simulink model "sim_new_traj_only_att_ctrl"  (R2020a)
settings: Solver=ode4  StartTime=0.0  StopTime=30.0  FixedStep=0.01  RelTol=1e-3
values from neighbouring files (symbols this model uses):
  beta_Phi_1 = pp0 * cal_frac_squ( 3, p_p0_plus_1, q_p0_plus_1 )                          * cal_frac_squ( eps_s_bar / pi, p_p0_min_2, q_p0_min_2 )                          / ( 2 * ( 2 * pp0 - 1 ) * tanh( gamma0 * ( eps_s_bar / pi ) / 2 ) )                          - ( cal_frac_squ( 3, p_p0_plus_1, q_p0_plus_1 ) * gamma0 / ( 4 * ( 2 * pp0 -1 ) ) )                          * cal_frac_squ( eps_s_bar / pi, p_p0_min_ ...(+136 chars)    [init_new_traj_only_att_ctrl.m]
  beta_Phi_2 = ( 1 - pp0 ) * cal_frac_squ( 3, p_p0_plus_1, q_p0_plus_1 )                          / ( 2 * ( 1 - 2 * pp0 ) * cal_frac_squ( eps_s_bar / pi, p_p0_0, q_p0_0 ) * tanh( gamma0 * ( eps_s_bar / pi ) / 2 ) )                          - ( cal_frac_squ( 3, p_p0_plus_1, q_p0_plus_1 ) * gamma0 / ( 4 * ( 1 - 2 * pp0 ) ) )                          * cal_frac_squ( eps_s_bar / pi, p_1_min_p0, q_1_min_p0 )          ...(+112 chars)    [init_new_traj_only_att_ctrl.m]
  c1_diff_sigma_bar_w = diag([12; 12; 12])    [init_new_traj_only_att_ctrl.m]
  c1_diff_ui = diag([25; 30; 20])    [init_new_traj_only_att_ctrl.m]
  c2_diff_sigma_bar_w = diag([12; 12; 12])    [init_new_traj_only_att_ctrl.m]
  c2_diff_ui = diag([50; 50; 10])    [init_new_traj_only_att_ctrl.m]
  c3_diff_sigma_bar_w = diag([15; 15; 15])    [init_new_traj_only_att_ctrl.m]
  c3_diff_ui = diag([15; 15; 10])    [init_new_traj_only_att_ctrl.m]
  c_w_1 = diag( [20; 15; 15] )    [init_new_traj_only_att_ctrl.m]
  c_w_2 = diag( [20; 15; 15] )    [init_new_traj_only_att_ctrl.m]
  c_w_3 = diag( [2; 2; 2] )    [init_new_traj_only_att_ctrl.m]
  cS0 = diag( [4.5; 4.5; 4.5] )    [init_new_traj_only_att_ctrl.m]
  dw_aa_t = 0.2 * ones(3, 5) + ( 1.0 - 0.2 ) * rand(3, 5)    [init_new_traj_only_att_ctrl.m]
  dw_ff_t = [ 0.4 * ones(1, 5) + ( 1.0 - 0.4 ) * rand(1, 5);                      0.4 * ones(1, 5) + ( 1.0 - 0.4 ) * rand(1, 5);                      0.2 * ones(1, 5) + ( 0.6 - 0.2 ) * rand(1, 5) ]    [init_new_traj_only_att_ctrl.m]
  dw_phi_t = ( - pi / 2 ) * ones(3, 5) + ( pi / 2 - ( - pi / 2 ) ) * rand(3, 5)    [init_new_traj_only_att_ctrl.m]
  dwci_init = zeros(3,5)    [init_new_traj_only_att_ctrl.m]
  eps_s_bar_div_pi = eps_s_bar / pi    (= 0.03)    [init_new_traj_only_att_ctrl.m]
  gamma0 = 20    [init_new_traj_only_att_ctrl.m]
  h1w = diag([20.0; 20.0; 20.0])    [init_new_traj_only_att_ctrl.m]
  h2w = diag([30.0; 35.0; 35.0])    [init_new_traj_only_att_ctrl.m]
  h3w = diag([30.0; 25.0; 30.0])    [init_new_traj_only_att_ctrl.m]
  Ji = zeros(3,3,NF)    [init_new_traj_only_att_ctrl.m]
  k_J_0 = diag( [1; 1; 1] )    [init_new_traj_only_att_ctrl.m]
  Lamd_diff_sigma_bar_w = 0.8    [init_new_traj_only_att_ctrl.m]
  Lamd_diff_ui = 0.8    [init_new_traj_only_att_ctrl.m]
  mu_c_theta = 100    [init_new_traj_only_att_ctrl.m]
  mu_d_w = 100    [init_new_traj_only_att_ctrl.m]
  pos0 = zeros(3, 1)    [init_new_traj_only_att_ctrl.m]
  pp0 = 8 / 11    (= 0.727272727273)    [init_new_traj_only_att_ctrl.m]
  PZ0 = P0(3)    [init_new_traj_only_att_ctrl.m]
  PZ1 = 10    [init_new_traj_only_att_ctrl.m]
  Qci_init = repmat([1;0;0;0],1,NF)    [init_new_traj_only_att_ctrl.m]
  R0 = 4    [init_new_traj_only_att_ctrl.m]
  R1 = 8    [init_new_traj_only_att_ctrl.m]
  Rci_init = zeros(3,3,NF)    [init_new_traj_only_att_ctrl.m]
  Ri_init = zeros(3,3,NF)    [init_new_traj_only_att_ctrl.m]
  Rx2 = 10    [init_new_traj_only_att_ctrl.m]
  Ry2 = 6    [init_new_traj_only_att_ctrl.m]
  Rz2 = 4    [init_new_traj_only_att_ctrl.m]
  T0 = 0    [init_new_traj_only_att_ctrl.m]
  T1 = tseq1    (= 10)    [init_new_traj_only_att_ctrl.m]
  T2 = tseq1 + tseq12 + tseq2    (= 30)    [init_new_traj_only_att_ctrl.m]
  thr_p_plus_1 = cal_frac_squ( 3, p_p0_plus_1, q_p0_plus_1 )    [init_new_traj_only_att_ctrl.m]
  ui_init = zeros(3,NF)    [init_new_traj_only_att_ctrl.m]
  vel0 = zeros(3, 1)    [init_new_traj_only_att_ctrl.m]
  wci_init = zeros(3,5)    [init_new_traj_only_att_ctrl.m]
  zeta_diff_sigma_bar_w = 0.3    [init_new_traj_only_att_ctrl.m]
  zeta_diff_ui = 0.05    [init_new_traj_only_att_ctrl.m]
undefined symbols (not defined in the file or in its folder): cal_frac_squ, p_2_p0, p_alfaw1, p_alfaw2, p_beta_w_1, p_beta_w_2, p_p0_min_1, p_p0_plus_1, q_2_p0, q_alfaw1, q_alfaw2, q_beta_w_1, q_beta_w_2, q_p0_min_1, q_p0_plus_1, Qei_init, Qi_init, Rei_init, V_Phi_Rei_init, wei_init, wi_init
(part 2 of 5)

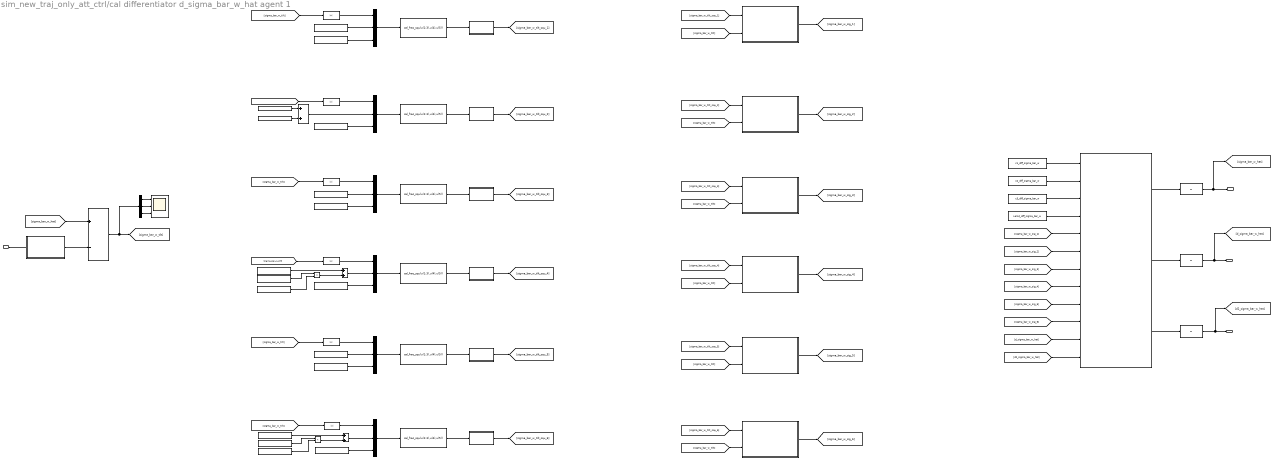
== system sim_new_traj_only_att_ctrl/cal differentiator d_sigma_bar_w_hat agent 1 ==
  x : Inport
  Abs{,1..5} (6 alike) : Abs
  Add : Sum
  Add1 : Sum
  Add2 : Sum
  Add3 : Sum  Inputs=+-
  Constant : Constant  Value=0
  Constant{97,100,105,107,109} (5 alike) : Constant
  Constant{98..99,101,108,110..111} (6 alike) : Constant  Value=3
  Constant102 : Constant  Value=2
  Constant103 : Constant  Value=c1_diff_sigma_bar_w
  Constant104 : Constant  Value=c2_diff_sigma_bar_w
  Constant106 : Constant  Value=c3_diff_sigma_bar_w
  Constant112 : Constant  Value=2
  Constant113 : Constant  Value=Lamd_diff_sigma_bar_w
  Constant161 : Constant  Value=zeta_diff_sigma_bar_w
  Constant162 : Constant  Value=zeta_diff_sigma_bar_w
  Constant163 : Constant  Value=zeta_diff_sigma_bar_w
  Demux2 : Demux  Outputs=3
  Integrator2 : Integrator  InitialCondition=zeros(3,1)
  Integrator3 : Integrator  InitialCondition=zeros(3,1)
  Integrator4 : Integrator  InitialCondition=zeros(3,1)
  Interpreted MATLAB Function{,20..24} (6 alike) : MATLABFcn  MATLABFcn=cal_frac_squ(u(1:3),u(4),u(5))
  Mux{19..24} (6 alike) : Mux  Inputs=3
  Product : Product
  Product1 : Product
  cal differentiator : MATLAB Function  TreatAsAtomicUnit=on
  cal sig : MATLAB Function  TreatAsAtomicUnit=on
  cal sig1 : MATLAB Function  TreatAsAtomicUnit=on
  cal sig2 : MATLAB Function  TreatAsAtomicUnit=on
  cal sig3 : MATLAB Function  TreatAsAtomicUnit=on
  cal sig4 : MATLAB Function  TreatAsAtomicUnit=on
  cal sig5 : MATLAB Function  TreatAsAtomicUnit=on
  choose sigma_bar_w : MATLAB Function  TreatAsAtomicUnit=on
  sigma_bar_w_tilt : Scope  NumInputPorts=3
  trans to column20 : MATLAB Function  TreatAsAtomicUnit=on
  trans to column21 : MATLAB Function  TreatAsAtomicUnit=on
  trans to column22 : MATLAB Function  TreatAsAtomicUnit=on
  trans to column23 : MATLAB Function  TreatAsAtomicUnit=on
  trans to column24 : MATLAB Function  TreatAsAtomicUnit=on
  trans to column25 : MATLAB Function  TreatAsAtomicUnit=on
  Out1 : Outport
  Out2 : Outport  Port=2
  Out3 : Outport  Port=3
  wires:
  Abs/1 -> Mux22/1
  [sigma_bar_w_tilt] -> cal sig/2(y)
  cal sig1/1(z) -> [sigma_bar_w_sig_2]
  [d2_sigma_bar_w_hat] -> cal differentiator/12(d2_sigma_bar_v_hat)
  trans to column23/1(y) -> [sigma_bar_w_tilt_squ_3]
  Add/1 -> Mux21/2
  Demux2/1 -> sigma_bar_w_tilt/1
  [sigma_bar_w_tilt] -> cal sig4/2(y)
  Product1/1 -> Add2/2
  Add2/1 -> Mux19/2
  [d_sigma_bar_w_hat] -> cal differentiator/11("d_sigma_bar_v_hat ")
  [sigma_bar_w_sig_3] -> cal differentiator/7(sigma_bar_v_sig_3)
  trans to column24/1(y) -> [sigma_bar_w_tilt_squ_4]
  Constant107/1 -> Mux21/3
  [sigma_bar_w_sig_5] -> cal differentiator/9(sigma_bar_v_sig_5)
  Constant97/1 -> Mux22/3
  cal sig/1(z) -> [sigma_bar_w_sig_1]
  trans to column22/1(y) -> [sigma_bar_w_tilt_squ_1]
  [sigma_bar_w_tilt_squ_3] -> cal sig2/1(x)
  [sigma_bar_w_tilt] -> Abs3/1
  Interpreted MATLAB Function24/1 -> trans to column25/1(x)
  [sigma_bar_w_sig_1] -> cal differentiator/5(sigma_bar_v_sig_1)
  cal differentiator/1(d_sigma_bar_v_hat) -> Integrator2/1
  Constant110/1 -> Mux24/3
  cal sig5/1(z) -> [sigma_bar_w_sig_5]
  [sigma_bar_w_tilt] -> Abs4/1
  Demux2/3 -> sigma_bar_w_tilt/3
  cal sig2/1(z) -> [sigma_bar_w_sig_3]
  Constant112/1 -> Product/1
  Constant/1 -> Mux22/2
  cal differentiator/3(d_d2sigma_bar_v_hat) -> Integrator4/1
  Abs3/1 -> Mux24/1
  trans to column21/1(y) -> [sigma_bar_w_tilt_squ_2]
  Constant99/1 -> Add2/1
  Constant103/1 -> cal differentiator/1(c1)
  Mux19/1 -> Interpreted MATLAB Function24/1
  [sigma_bar_w_tilt_squ_6] -> cal sig3/1(x)
  Constant106/1 -> cal differentiator/3(c3)
  [sigma_bar_w_tilt] -> Abs2/1
  [sigma_bar_w_tilt_squ_2] -> cal sig1/1(x)
  Constant162/1 -> Product/2
  Product/1 -> Add1/2
  [sigma_bar_w_sig_4] -> cal differentiator/8(sigma_bar_v_sig_4)
  [sigma_bar_w_hat] -> Add3/1
  Constant102/1 -> Mux20/2
  Add3/1 -> Demux2/1, [sigma_bar_w_tilt]
  cal differentiator/2(d_dsigma_bar_v_hat) -> Integrator3/1
  [sigma_bar_w_tilt] -> Abs5/1
  [sigma_bar_w_tilt] -> cal sig2/2(y)
  [sigma_bar_w_sig_6] -> cal differentiator/10(sigma_bar_v_sig_6)
  trans to column20/1(y) -> [sigma_bar_w_tilt_squ_5]
  Constant104/1 -> cal differentiator/2(c2)
  Constant101/1 -> Mux20/3
  Mux22/1 -> Interpreted MATLAB Function/1
  Constant163/1 -> Product1/2
  Abs2/1 -> Mux23/1
  Interpreted MATLAB Function21/1 -> trans to column21/1(x)
  Interpreted MATLAB Function23/1 -> trans to column24/1(x)
  Mux23/1 -> Interpreted MATLAB Function22/1
  cal sig3/1(z) -> [sigma_bar_w_sig_6]
  Abs4/1 -> Mux19/1
  trans to column25/1(y) -> [sigma_bar_w_tilt_squ_6]
  Constant113/1 -> cal differentiator/4(chi_t)
  choose sigma_bar_w/1(y) -> Add3/2
  Interpreted MATLAB Function/1 -> trans to column22/1(x)
  Interpreted MATLAB Function20/1 -> trans to column20/1(x)
  Constant108/1 -> Mux23/3
  [sigma_bar_w_sig_2] -> cal differentiator/6(sigma_bar_v_sig_2)
  [sigma_bar_w_tilt] -> cal sig1/2(y)
  [sigma_bar_w_tilt_squ_1] -> cal sig/1(x)
  Constant100/1 -> Product1/1
  Abs1/1 -> Mux21/1
  Demux2/2 -> sigma_bar_w_tilt/2
  Integrator4/1 -> [d2_sigma_bar_w_hat], Out3/1
  [sigma_bar_w_tilt_squ_4] -> cal sig4/1(x)
  Abs5/1 -> Mux20/1
  Constant98/1 -> Mux19/3
  Constant111/1 -> Add1/1
  [sigma_bar_w_tilt] -> cal sig5/2(y)
  Constant109/1 -> Mux23/2
  [sigma_bar_w_tilt] -> Abs/1
  Mux24/1 -> Interpreted MATLAB Function23/1
  [sigma_bar_w_tilt] -> Abs1/1
  [sigma_bar_w_tilt_squ_5] -> cal sig5/1(x)
  Add1/1 -> Mux24/2
  cal sig4/1(z) -> [sigma_bar_w_sig_4]
  Constant161/1 -> Add/2
  [sigma_bar_w_tilt] -> cal sig3/2(y)
  Mux21/1 -> Interpreted MATLAB Function21/1
  Interpreted MATLAB Function22/1 -> trans to column23/1(x)
  Mux20/1 -> Interpreted MATLAB Function20/1
  x/1 -> choose sigma_bar_w/1(x)
  Constant105/1 -> Add/1
  Integrator2/1 -> [sigma_bar_w_hat], Out1/1
  Integrator3/1 -> [d_sigma_bar_w_hat], Out2/1

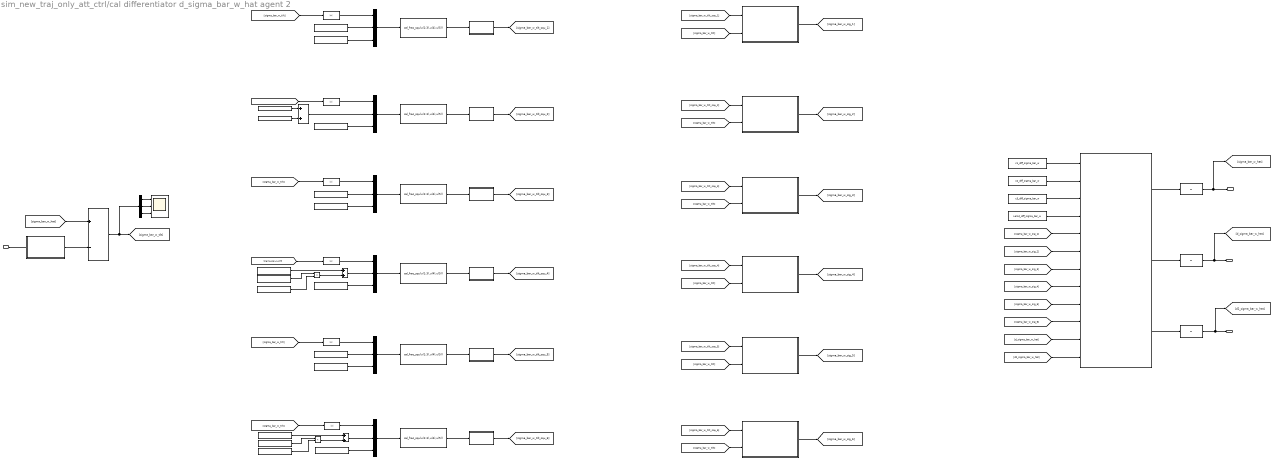
== system sim_new_traj_only_att_ctrl/cal differentiator d_sigma_bar_w_hat agent 2 ==
  x : Inport
  Abs{,1..5} (6 alike) : Abs
  Add : Sum
  Add1 : Sum
  Add2 : Sum
  Add3 : Sum  Inputs=+-
  Constant : Constant  Value=0
  Constant{97,100,105,107,109} (5 alike) : Constant
  Constant{98..99,101,108,110..111} (6 alike) : Constant  Value=3
  Constant102 : Constant  Value=2
  Constant103 : Constant  Value=c1_diff_sigma_bar_w
  Constant104 : Constant  Value=c2_diff_sigma_bar_w
  Constant106 : Constant  Value=c3_diff_sigma_bar_w
  Constant112 : Constant  Value=2
  Constant113 : Constant  Value=Lamd_diff_sigma_bar_w
  Constant161 : Constant  Value=zeta_diff_sigma_bar_w
  Constant162 : Constant  Value=zeta_diff_sigma_bar_w
  Constant163 : Constant  Value=zeta_diff_sigma_bar_w
  Demux2 : Demux  Outputs=3
  Integrator2 : Integrator  InitialCondition=zeros(3,1)
  Integrator3 : Integrator  InitialCondition=zeros(3,1)
  Integrator4 : Integrator  InitialCondition=zeros(3,1)
  Interpreted MATLAB Function{,20..24} (6 alike) : MATLABFcn  MATLABFcn=cal_frac_squ(u(1:3),u(4),u(5))
  Mux{19..24} (6 alike) : Mux  Inputs=3
  Product : Product
  Product1 : Product
  cal differentiator : MATLAB Function  TreatAsAtomicUnit=on
  cal sig : MATLAB Function  TreatAsAtomicUnit=on
  cal sig1 : MATLAB Function  TreatAsAtomicUnit=on
  cal sig2 : MATLAB Function  TreatAsAtomicUnit=on
  cal sig3 : MATLAB Function  TreatAsAtomicUnit=on
  cal sig4 : MATLAB Function  TreatAsAtomicUnit=on
  cal sig5 : MATLAB Function  TreatAsAtomicUnit=on
  choose sigma_bar_w : MATLAB Function  TreatAsAtomicUnit=on
  sigma_bar_w_tilt : Scope  NumInputPorts=3
  trans to column20 : MATLAB Function  TreatAsAtomicUnit=on
  trans to column21 : MATLAB Function  TreatAsAtomicUnit=on
  trans to column22 : MATLAB Function  TreatAsAtomicUnit=on
  trans to column23 : MATLAB Function  TreatAsAtomicUnit=on
  trans to column24 : MATLAB Function  TreatAsAtomicUnit=on
  trans to column25 : MATLAB Function  TreatAsAtomicUnit=on
  Out1 : Outport
  Out2 : Outport  Port=2
  Out3 : Outport  Port=3
  wires:
  Abs/1 -> Mux22/1
  [sigma_bar_w_tilt] -> cal sig/2(y)
  cal sig1/1(z) -> [sigma_bar_w_sig_2]
  [d2_sigma_bar_w_hat] -> cal differentiator/12(d2_sigma_bar_v_hat)
  trans to column23/1(y) -> [sigma_bar_w_tilt_squ_3]
  Add/1 -> Mux21/2
  Demux2/1 -> sigma_bar_w_tilt/1
  [sigma_bar_w_tilt] -> cal sig4/2(y)
  Product1/1 -> Add2/2
  Add2/1 -> Mux19/2
  [d_sigma_bar_w_hat] -> cal differentiator/11("d_sigma_bar_v_hat ")
  [sigma_bar_w_sig_3] -> cal differentiator/7(sigma_bar_v_sig_3)
  trans to column24/1(y) -> [sigma_bar_w_tilt_squ_4]
  Constant107/1 -> Mux21/3
  [sigma_bar_w_sig_5] -> cal differentiator/9(sigma_bar_v_sig_5)
  Constant97/1 -> Mux22/3
  cal sig/1(z) -> [sigma_bar_w_sig_1]
  trans to column22/1(y) -> [sigma_bar_w_tilt_squ_1]
  [sigma_bar_w_tilt_squ_3] -> cal sig2/1(x)
  [sigma_bar_w_tilt] -> Abs3/1
  Interpreted MATLAB Function24/1 -> trans to column25/1(x)
  [sigma_bar_w_sig_1] -> cal differentiator/5(sigma_bar_v_sig_1)
  cal differentiator/1(d_sigma_bar_v_hat) -> Integrator2/1
  Constant110/1 -> Mux24/3
  cal sig5/1(z) -> [sigma_bar_w_sig_5]
  [sigma_bar_w_tilt] -> Abs4/1
  Demux2/3 -> sigma_bar_w_tilt/3
  cal sig2/1(z) -> [sigma_bar_w_sig_3]
  Constant112/1 -> Product/1
  Constant/1 -> Mux22/2
  cal differentiator/3(d_d2sigma_bar_v_hat) -> Integrator4/1
  Abs3/1 -> Mux24/1
  trans to column21/1(y) -> [sigma_bar_w_tilt_squ_2]
  Constant99/1 -> Add2/1
  Constant103/1 -> cal differentiator/1(c1)
  Mux19/1 -> Interpreted MATLAB Function24/1
  [sigma_bar_w_tilt_squ_6] -> cal sig3/1(x)
  Constant106/1 -> cal differentiator/3(c3)
  [sigma_bar_w_tilt] -> Abs2/1
  [sigma_bar_w_tilt_squ_2] -> cal sig1/1(x)
  Constant162/1 -> Product/2
  Product/1 -> Add1/2
  [sigma_bar_w_sig_4] -> cal differentiator/8(sigma_bar_v_sig_4)
  [sigma_bar_w_hat] -> Add3/1
  Constant102/1 -> Mux20/2
  Add3/1 -> Demux2/1, [sigma_bar_w_tilt]
  cal differentiator/2(d_dsigma_bar_v_hat) -> Integrator3/1
  [sigma_bar_w_tilt] -> Abs5/1
  [sigma_bar_w_tilt] -> cal sig2/2(y)
  [sigma_bar_w_sig_6] -> cal differentiator/10(sigma_bar_v_sig_6)
  trans to column20/1(y) -> [sigma_bar_w_tilt_squ_5]
  Constant104/1 -> cal differentiator/2(c2)
  Constant101/1 -> Mux20/3
  Mux22/1 -> Interpreted MATLAB Function/1
  Constant163/1 -> Product1/2
  Abs2/1 -> Mux23/1
  Interpreted MATLAB Function21/1 -> trans to column21/1(x)
  Interpreted MATLAB Function23/1 -> trans to column24/1(x)
  Mux23/1 -> Interpreted MATLAB Function22/1
  cal sig3/1(z) -> [sigma_bar_w_sig_6]
  Abs4/1 -> Mux19/1
  trans to column25/1(y) -> [sigma_bar_w_tilt_squ_6]
  Constant113/1 -> cal differentiator/4(chi_t)
  choose sigma_bar_w/1(y) -> Add3/2
  Interpreted MATLAB Function/1 -> trans to column22/1(x)
  Interpreted MATLAB Function20/1 -> trans to column20/1(x)
  Constant108/1 -> Mux23/3
  [sigma_bar_w_sig_2] -> cal differentiator/6(sigma_bar_v_sig_2)
  [sigma_bar_w_tilt] -> cal sig1/2(y)
  [sigma_bar_w_tilt_squ_1] -> cal sig/1(x)
  Constant100/1 -> Product1/1
  Abs1/1 -> Mux21/1
  Demux2/2 -> sigma_bar_w_tilt/2
  Integrator4/1 -> [d2_sigma_bar_w_hat], Out3/1
  [sigma_bar_w_tilt_squ_4] -> cal sig4/1(x)
  Abs5/1 -> Mux20/1
  Constant98/1 -> Mux19/3
  Constant111/1 -> Add1/1
  [sigma_bar_w_tilt] -> cal sig5/2(y)
  Constant109/1 -> Mux23/2
  [sigma_bar_w_tilt] -> Abs/1
  Mux24/1 -> Interpreted MATLAB Function23/1
  [sigma_bar_w_tilt] -> Abs1/1
  [sigma_bar_w_tilt_squ_5] -> cal sig5/1(x)
  Add1/1 -> Mux24/2
  cal sig4/1(z) -> [sigma_bar_w_sig_4]
  Constant161/1 -> Add/2
  [sigma_bar_w_tilt] -> cal sig3/2(y)
  Mux21/1 -> Interpreted MATLAB Function21/1
  Interpreted MATLAB Function22/1 -> trans to column23/1(x)
  Mux20/1 -> Interpreted MATLAB Function20/1
  x/1 -> choose sigma_bar_w/1(x)
  Constant105/1 -> Add/1
  Integrator2/1 -> [sigma_bar_w_hat], Out1/1
  Integrator3/1 -> [d_sigma_bar_w_hat], Out2/1

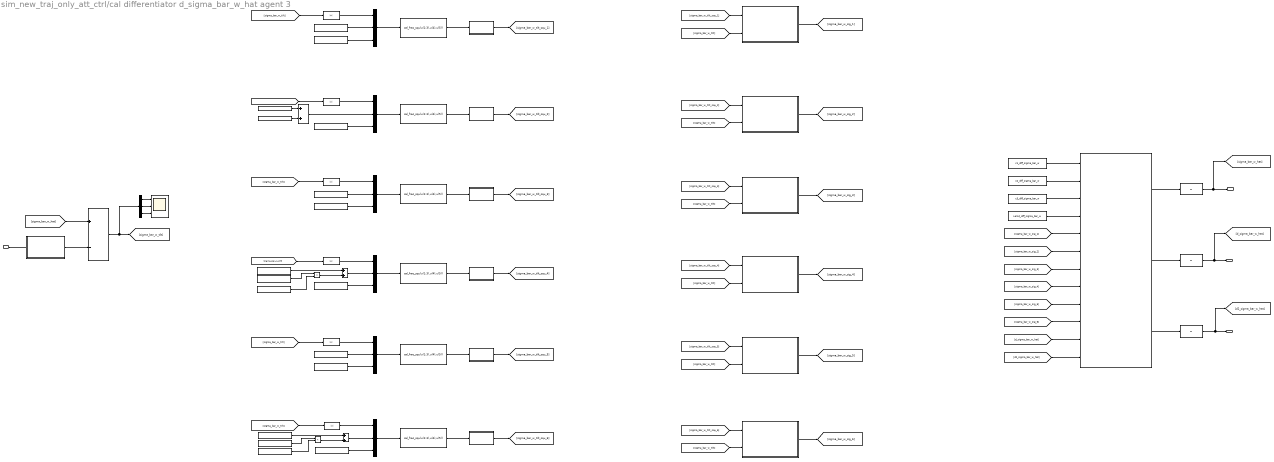
== system sim_new_traj_only_att_ctrl/cal differentiator d_sigma_bar_w_hat agent 3 ==
  x : Inport
  Abs{,1..5} (6 alike) : Abs
  Add : Sum
  Add1 : Sum
  Add2 : Sum
  Add3 : Sum  Inputs=+-
  Constant : Constant  Value=0
  Constant{97,100,105,107,109} (5 alike) : Constant
  Constant{98..99,101,108,110..111} (6 alike) : Constant  Value=3
  Constant102 : Constant  Value=2
  Constant103 : Constant  Value=c1_diff_sigma_bar_w
  Constant104 : Constant  Value=c2_diff_sigma_bar_w
  Constant106 : Constant  Value=c3_diff_sigma_bar_w
  Constant112 : Constant  Value=2
  Constant113 : Constant  Value=Lamd_diff_sigma_bar_w
  Constant161 : Constant  Value=zeta_diff_sigma_bar_w
  Constant162 : Constant  Value=zeta_diff_sigma_bar_w
  Constant163 : Constant  Value=zeta_diff_sigma_bar_w
  Demux2 : Demux  Outputs=3
  Integrator2 : Integrator  InitialCondition=zeros(3,1)
  Integrator3 : Integrator  InitialCondition=zeros(3,1)
  Integrator4 : Integrator  InitialCondition=zeros(3,1)
  Interpreted MATLAB Function{,20..24} (6 alike) : MATLABFcn  MATLABFcn=cal_frac_squ(u(1:3),u(4),u(5))
  Mux{19..24} (6 alike) : Mux  Inputs=3
  Product : Product
  Product1 : Product
  cal differentiator : MATLAB Function  TreatAsAtomicUnit=on
  cal sig : MATLAB Function  TreatAsAtomicUnit=on
  cal sig1 : MATLAB Function  TreatAsAtomicUnit=on
  cal sig2 : MATLAB Function  TreatAsAtomicUnit=on
  cal sig3 : MATLAB Function  TreatAsAtomicUnit=on
  cal sig4 : MATLAB Function  TreatAsAtomicUnit=on
  cal sig5 : MATLAB Function  TreatAsAtomicUnit=on
  choose sigma_bar_w : MATLAB Function  TreatAsAtomicUnit=on
  sigma_bar_w_tilt : Scope  NumInputPorts=3
  trans to column20 : MATLAB Function  TreatAsAtomicUnit=on
  trans to column21 : MATLAB Function  TreatAsAtomicUnit=on
  trans to column22 : MATLAB Function  TreatAsAtomicUnit=on
  trans to column23 : MATLAB Function  TreatAsAtomicUnit=on
  trans to column24 : MATLAB Function  TreatAsAtomicUnit=on
  trans to column25 : MATLAB Function  TreatAsAtomicUnit=on
  Out1 : Outport
  Out2 : Outport  Port=2
  Out3 : Outport  Port=3
  wires:
  Abs/1 -> Mux22/1
  [sigma_bar_w_tilt] -> cal sig/2(y)
  cal sig1/1(z) -> [sigma_bar_w_sig_2]
  [d2_sigma_bar_w_hat] -> cal differentiator/12(d2_sigma_bar_v_hat)
  trans to column23/1(y) -> [sigma_bar_w_tilt_squ_3]
  Add/1 -> Mux21/2
  Demux2/1 -> sigma_bar_w_tilt/1
  [sigma_bar_w_tilt] -> cal sig4/2(y)
  Product1/1 -> Add2/2
  Add2/1 -> Mux19/2
  [d_sigma_bar_w_hat] -> cal differentiator/11("d_sigma_bar_v_hat ")
  [sigma_bar_w_sig_3] -> cal differentiator/7(sigma_bar_v_sig_3)
  trans to column24/1(y) -> [sigma_bar_w_tilt_squ_4]
  Constant107/1 -> Mux21/3
  [sigma_bar_w_sig_5] -> cal differentiator/9(sigma_bar_v_sig_5)
  Constant97/1 -> Mux22/3
  cal sig/1(z) -> [sigma_bar_w_sig_1]
  trans to column22/1(y) -> [sigma_bar_w_tilt_squ_1]
  [sigma_bar_w_tilt_squ_3] -> cal sig2/1(x)
  [sigma_bar_w_tilt] -> Abs3/1
  Interpreted MATLAB Function24/1 -> trans to column25/1(x)
  [sigma_bar_w_sig_1] -> cal differentiator/5(sigma_bar_v_sig_1)
  cal differentiator/1(d_sigma_bar_v_hat) -> Integrator2/1
  Constant110/1 -> Mux24/3
  cal sig5/1(z) -> [sigma_bar_w_sig_5]
  [sigma_bar_w_tilt] -> Abs4/1
  Demux2/3 -> sigma_bar_w_tilt/3
  cal sig2/1(z) -> [sigma_bar_w_sig_3]
  Constant112/1 -> Product/1
  Constant/1 -> Mux22/2
  cal differentiator/3(d_d2sigma_bar_v_hat) -> Integrator4/1
  Abs3/1 -> Mux24/1
  trans to column21/1(y) -> [sigma_bar_w_tilt_squ_2]
  Constant99/1 -> Add2/1
  Constant103/1 -> cal differentiator/1(c1)
  Mux19/1 -> Interpreted MATLAB Function24/1
  [sigma_bar_w_tilt_squ_6] -> cal sig3/1(x)
  Constant106/1 -> cal differentiator/3(c3)
  [sigma_bar_w_tilt] -> Abs2/1
  [sigma_bar_w_tilt_squ_2] -> cal sig1/1(x)
  Constant162/1 -> Product/2
  Product/1 -> Add1/2
  [sigma_bar_w_sig_4] -> cal differentiator/8(sigma_bar_v_sig_4)
  [sigma_bar_w_hat] -> Add3/1
  Constant102/1 -> Mux20/2
  Add3/1 -> Demux2/1, [sigma_bar_w_tilt]
  cal differentiator/2(d_dsigma_bar_v_hat) -> Integrator3/1
  [sigma_bar_w_tilt] -> Abs5/1
  [sigma_bar_w_tilt] -> cal sig2/2(y)
  [sigma_bar_w_sig_6] -> cal differentiator/10(sigma_bar_v_sig_6)
  trans to column20/1(y) -> [sigma_bar_w_tilt_squ_5]
  Constant104/1 -> cal differentiator/2(c2)
  Constant101/1 -> Mux20/3
  Mux22/1 -> Interpreted MATLAB Function/1
  Constant163/1 -> Product1/2
  Abs2/1 -> Mux23/1
  Interpreted MATLAB Function21/1 -> trans to column21/1(x)
  Interpreted MATLAB Function23/1 -> trans to column24/1(x)
  Mux23/1 -> Interpreted MATLAB Function22/1
  cal sig3/1(z) -> [sigma_bar_w_sig_6]
  Abs4/1 -> Mux19/1
  trans to column25/1(y) -> [sigma_bar_w_tilt_squ_6]
  Constant113/1 -> cal differentiator/4(chi_t)
  choose sigma_bar_w/1(y) -> Add3/2
  Interpreted MATLAB Function/1 -> trans to column22/1(x)
  Interpreted MATLAB Function20/1 -> trans to column20/1(x)
  Constant108/1 -> Mux23/3
  [sigma_bar_w_sig_2] -> cal differentiator/6(sigma_bar_v_sig_2)
  [sigma_bar_w_tilt] -> cal sig1/2(y)
  [sigma_bar_w_tilt_squ_1] -> cal sig/1(x)
  Constant100/1 -> Product1/1
  Abs1/1 -> Mux21/1
  Demux2/2 -> sigma_bar_w_tilt/2
  Integrator4/1 -> [d2_sigma_bar_w_hat], Out3/1
  [sigma_bar_w_tilt_squ_4] -> cal sig4/1(x)
  Abs5/1 -> Mux20/1
  Constant98/1 -> Mux19/3
  Constant111/1 -> Add1/1
  [sigma_bar_w_tilt] -> cal sig5/2(y)
  Constant109/1 -> Mux23/2
  [sigma_bar_w_tilt] -> Abs/1
  Mux24/1 -> Interpreted MATLAB Function23/1
  [sigma_bar_w_tilt] -> Abs1/1
  [sigma_bar_w_tilt_squ_5] -> cal sig5/1(x)
  Add1/1 -> Mux24/2
  cal sig4/1(z) -> [sigma_bar_w_sig_4]
  Constant161/1 -> Add/2
  [sigma_bar_w_tilt] -> cal sig3/2(y)
  Mux21/1 -> Interpreted MATLAB Function21/1
  Interpreted MATLAB Function22/1 -> trans to column23/1(x)
  Mux20/1 -> Interpreted MATLAB Function20/1
  x/1 -> choose sigma_bar_w/1(x)
  Constant105/1 -> Add/1
  Integrator2/1 -> [sigma_bar_w_hat], Out1/1
  Integrator3/1 -> [d_sigma_bar_w_hat], Out2/1

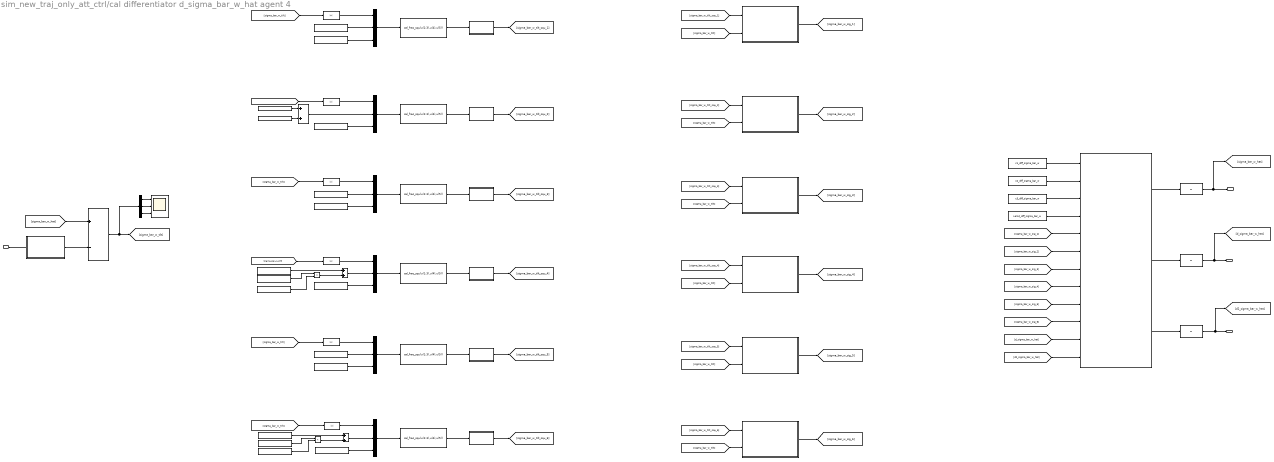
== system sim_new_traj_only_att_ctrl/cal differentiator d_sigma_bar_w_hat agent 4 ==
  x : Inport
  Abs{,1..5} (6 alike) : Abs
  Add : Sum
  Add1 : Sum
  Add2 : Sum
  Add3 : Sum  Inputs=+-
  Constant : Constant  Value=0
  Constant{97,100,105,107,109} (5 alike) : Constant
  Constant{98..99,101,108,110..111} (6 alike) : Constant  Value=3
  Constant102 : Constant  Value=2
  Constant103 : Constant  Value=c1_diff_sigma_bar_w
  Constant104 : Constant  Value=c2_diff_sigma_bar_w
  Constant106 : Constant  Value=c3_diff_sigma_bar_w
  Constant112 : Constant  Value=2
  Constant113 : Constant  Value=Lamd_diff_sigma_bar_w
  Constant161 : Constant  Value=zeta_diff_sigma_bar_w
  Constant162 : Constant  Value=zeta_diff_sigma_bar_w
  Constant163 : Constant  Value=zeta_diff_sigma_bar_w
  Demux2 : Demux  Outputs=3
  Integrator2 : Integrator  InitialCondition=zeros(3,1)
  Integrator3 : Integrator  InitialCondition=zeros(3,1)
  Integrator4 : Integrator  InitialCondition=zeros(3,1)
  Interpreted MATLAB Function{,20..24} (6 alike) : MATLABFcn  MATLABFcn=cal_frac_squ(u(1:3),u(4),u(5))
  Mux{19..24} (6 alike) : Mux  Inputs=3
  Product : Product
  Product1 : Product
  cal differentiator : MATLAB Function  TreatAsAtomicUnit=on
  cal sig : MATLAB Function  TreatAsAtomicUnit=on
  cal sig1 : MATLAB Function  TreatAsAtomicUnit=on
  cal sig2 : MATLAB Function  TreatAsAtomicUnit=on
  cal sig3 : MATLAB Function  TreatAsAtomicUnit=on
  cal sig4 : MATLAB Function  TreatAsAtomicUnit=on
  cal sig5 : MATLAB Function  TreatAsAtomicUnit=on
  choose sigma_bar_w : MATLAB Function  TreatAsAtomicUnit=on
  sigma_bar_w_tilt : Scope  NumInputPorts=3
  trans to column20 : MATLAB Function  TreatAsAtomicUnit=on
  trans to column21 : MATLAB Function  TreatAsAtomicUnit=on
  trans to column22 : MATLAB Function  TreatAsAtomicUnit=on
  trans to column23 : MATLAB Function  TreatAsAtomicUnit=on
  trans to column24 : MATLAB Function  TreatAsAtomicUnit=on
  trans to column25 : MATLAB Function  TreatAsAtomicUnit=on
  Out1 : Outport
  Out2 : Outport  Port=2
  Out3 : Outport  Port=3
  wires:
  Abs/1 -> Mux22/1
  [sigma_bar_w_tilt] -> cal sig/2(y)
  cal sig1/1(z) -> [sigma_bar_w_sig_2]
  [d2_sigma_bar_w_hat] -> cal differentiator/12(d2_sigma_bar_v_hat)
  trans to column23/1(y) -> [sigma_bar_w_tilt_squ_3]
  Add/1 -> Mux21/2
  Demux2/1 -> sigma_bar_w_tilt/1
  [sigma_bar_w_tilt] -> cal sig4/2(y)
  Product1/1 -> Add2/2
  Add2/1 -> Mux19/2
  [d_sigma_bar_w_hat] -> cal differentiator/11("d_sigma_bar_v_hat ")
  [sigma_bar_w_sig_3] -> cal differentiator/7(sigma_bar_v_sig_3)
  trans to column24/1(y) -> [sigma_bar_w_tilt_squ_4]
  Constant107/1 -> Mux21/3
  [sigma_bar_w_sig_5] -> cal differentiator/9(sigma_bar_v_sig_5)
  Constant97/1 -> Mux22/3
  cal sig/1(z) -> [sigma_bar_w_sig_1]
  trans to column22/1(y) -> [sigma_bar_w_tilt_squ_1]
  [sigma_bar_w_tilt_squ_3] -> cal sig2/1(x)
  [sigma_bar_w_tilt] -> Abs3/1
  Interpreted MATLAB Function24/1 -> trans to column25/1(x)
  [sigma_bar_w_sig_1] -> cal differentiator/5(sigma_bar_v_sig_1)
  cal differentiator/1(d_sigma_bar_v_hat) -> Integrator2/1
  Constant110/1 -> Mux24/3
  cal sig5/1(z) -> [sigma_bar_w_sig_5]
  [sigma_bar_w_tilt] -> Abs4/1
  Demux2/3 -> sigma_bar_w_tilt/3
  cal sig2/1(z) -> [sigma_bar_w_sig_3]
  Constant112/1 -> Product/1
  Constant/1 -> Mux22/2
  cal differentiator/3(d_d2sigma_bar_v_hat) -> Integrator4/1
  Abs3/1 -> Mux24/1
  trans to column21/1(y) -> [sigma_bar_w_tilt_squ_2]
  Constant99/1 -> Add2/1
  Constant103/1 -> cal differentiator/1(c1)
  Mux19/1 -> Interpreted MATLAB Function24/1
  [sigma_bar_w_tilt_squ_6] -> cal sig3/1(x)
  Constant106/1 -> cal differentiator/3(c3)
  [sigma_bar_w_tilt] -> Abs2/1
  [sigma_bar_w_tilt_squ_2] -> cal sig1/1(x)
  Constant162/1 -> Product/2
  Product/1 -> Add1/2
  [sigma_bar_w_sig_4] -> cal differentiator/8(sigma_bar_v_sig_4)
  [sigma_bar_w_hat] -> Add3/1
  Constant102/1 -> Mux20/2
  Add3/1 -> Demux2/1, [sigma_bar_w_tilt]
  cal differentiator/2(d_dsigma_bar_v_hat) -> Integrator3/1
  [sigma_bar_w_tilt] -> Abs5/1
  [sigma_bar_w_tilt] -> cal sig2/2(y)
  [sigma_bar_w_sig_6] -> cal differentiator/10(sigma_bar_v_sig_6)
  trans to column20/1(y) -> [sigma_bar_w_tilt_squ_5]
  Constant104/1 -> cal differentiator/2(c2)
  Constant101/1 -> Mux20/3
  Mux22/1 -> Interpreted MATLAB Function/1
  Constant163/1 -> Product1/2
  Abs2/1 -> Mux23/1
  Interpreted MATLAB Function21/1 -> trans to column21/1(x)
  Interpreted MATLAB Function23/1 -> trans to column24/1(x)
  Mux23/1 -> Interpreted MATLAB Function22/1
  cal sig3/1(z) -> [sigma_bar_w_sig_6]
  Abs4/1 -> Mux19/1
  trans to column25/1(y) -> [sigma_bar_w_tilt_squ_6]
  Constant113/1 -> cal differentiator/4(chi_t)
  choose sigma_bar_w/1(y) -> Add3/2
  Interpreted MATLAB Function/1 -> trans to column22/1(x)
  Interpreted MATLAB Function20/1 -> trans to column20/1(x)
  Constant108/1 -> Mux23/3
  [sigma_bar_w_sig_2] -> cal differentiator/6(sigma_bar_v_sig_2)
  [sigma_bar_w_tilt] -> cal sig1/2(y)
  [sigma_bar_w_tilt_squ_1] -> cal sig/1(x)
  Constant100/1 -> Product1/1
  Abs1/1 -> Mux21/1
  Demux2/2 -> sigma_bar_w_tilt/2
  Integrator4/1 -> [d2_sigma_bar_w_hat], Out3/1
  [sigma_bar_w_tilt_squ_4] -> cal sig4/1(x)
  Abs5/1 -> Mux20/1
  Constant98/1 -> Mux19/3
  Constant111/1 -> Add1/1
  [sigma_bar_w_tilt] -> cal sig5/2(y)
  Constant109/1 -> Mux23/2
  [sigma_bar_w_tilt] -> Abs/1
  Mux24/1 -> Interpreted MATLAB Function23/1
  [sigma_bar_w_tilt] -> Abs1/1
  [sigma_bar_w_tilt_squ_5] -> cal sig5/1(x)
  Add1/1 -> Mux24/2
  cal sig4/1(z) -> [sigma_bar_w_sig_4]
  Constant161/1 -> Add/2
  [sigma_bar_w_tilt] -> cal sig3/2(y)
  Mux21/1 -> Interpreted MATLAB Function21/1
  Interpreted MATLAB Function22/1 -> trans to column23/1(x)
  Mux20/1 -> Interpreted MATLAB Function20/1
  x/1 -> choose sigma_bar_w/1(x)
  Constant105/1 -> Add/1
  Integrator2/1 -> [sigma_bar_w_hat], Out1/1
  Integrator3/1 -> [d_sigma_bar_w_hat], Out2/1

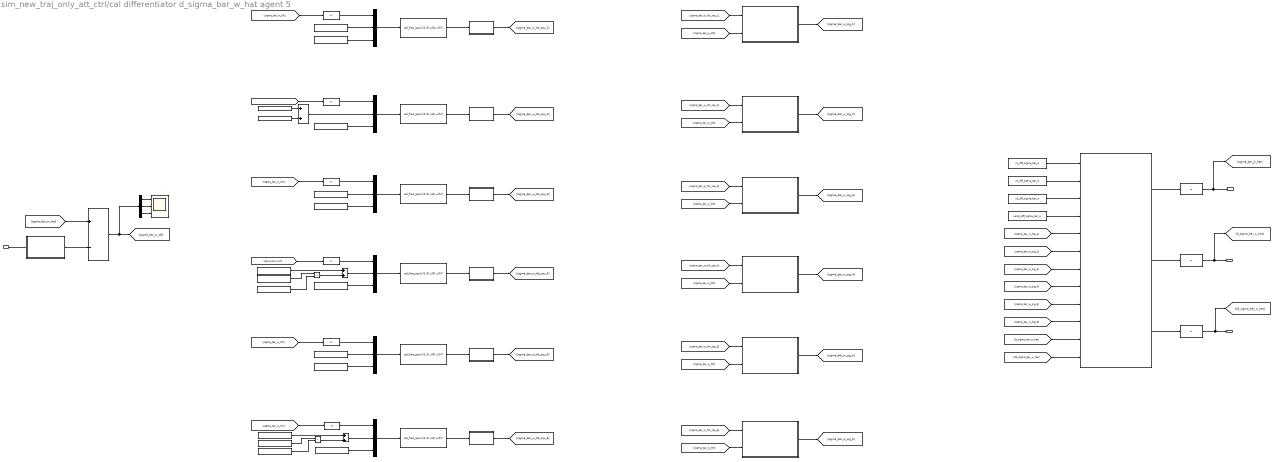
== system sim_new_traj_only_att_ctrl/cal differentiator d_sigma_bar_w_hat agent 5 ==
  x : Inport
  Abs{,1..5} (6 alike) : Abs
  Add : Sum
  Add1 : Sum
  Add2 : Sum
  Add3 : Sum  Inputs=+-
  Constant : Constant  Value=0
  Constant{97,100,105,107,109} (5 alike) : Constant
  Constant{98..99,101,108,110..111} (6 alike) : Constant  Value=3
  Constant102 : Constant  Value=2
  Constant103 : Constant  Value=c1_diff_sigma_bar_w
  Constant104 : Constant  Value=c2_diff_sigma_bar_w
  Constant106 : Constant  Value=c3_diff_sigma_bar_w
  Constant112 : Constant  Value=2
  Constant113 : Constant  Value=Lamd_diff_sigma_bar_w
  Constant161 : Constant  Value=zeta_diff_sigma_bar_w
  Constant162 : Constant  Value=zeta_diff_sigma_bar_w
  Constant163 : Constant  Value=zeta_diff_sigma_bar_w
  Demux2 : Demux  Outputs=3
  Integrator2 : Integrator  InitialCondition=zeros(3,1)
  Integrator3 : Integrator  InitialCondition=zeros(3,1)
  Integrator4 : Integrator  InitialCondition=zeros(3,1)
  Interpreted MATLAB Function{,20..24} (6 alike) : MATLABFcn  MATLABFcn=cal_frac_squ(u(1:3),u(4),u(5))
  Mux{19..24} (6 alike) : Mux  Inputs=3
  Product : Product
  Product1 : Product
  cal differentiator : MATLAB Function  TreatAsAtomicUnit=on
  cal sig : MATLAB Function  TreatAsAtomicUnit=on
  cal sig1 : MATLAB Function  TreatAsAtomicUnit=on
  cal sig2 : MATLAB Function  TreatAsAtomicUnit=on
  cal sig3 : MATLAB Function  TreatAsAtomicUnit=on
  cal sig4 : MATLAB Function  TreatAsAtomicUnit=on
  cal sig5 : MATLAB Function  TreatAsAtomicUnit=on
  choose sigma_bar_w : MATLAB Function  TreatAsAtomicUnit=on
  sigma_bar_w_tilt : Scope  NumInputPorts=3
  trans to column20 : MATLAB Function  TreatAsAtomicUnit=on
  trans to column21 : MATLAB Function  TreatAsAtomicUnit=on
  trans to column22 : MATLAB Function  TreatAsAtomicUnit=on
  trans to column23 : MATLAB Function  TreatAsAtomicUnit=on
  trans to column24 : MATLAB Function  TreatAsAtomicUnit=on
  trans to column25 : MATLAB Function  TreatAsAtomicUnit=on
  Out1 : Outport
  Out2 : Outport  Port=2
  Out3 : Outport  Port=3
  wires:
  Abs/1 -> Mux22/1
  [sigma_bar_w_tilt] -> cal sig/2(y)
  cal sig1/1(z) -> [sigma_bar_w_sig_2]
  [d2_sigma_bar_w_hat] -> cal differentiator/12(d2_sigma_bar_v_hat)
  trans to column23/1(y) -> [sigma_bar_w_tilt_squ_3]
  Add/1 -> Mux21/2
  Demux2/1 -> sigma_bar_w_tilt/1
  [sigma_bar_w_tilt] -> cal sig4/2(y)
  Product1/1 -> Add2/2
  Add2/1 -> Mux19/2
  [d_sigma_bar_w_hat] -> cal differentiator/11("d_sigma_bar_v_hat ")
  [sigma_bar_w_sig_3] -> cal differentiator/7(sigma_bar_v_sig_3)
  trans to column24/1(y) -> [sigma_bar_w_tilt_squ_4]
  Constant107/1 -> Mux21/3
  [sigma_bar_w_sig_5] -> cal differentiator/9(sigma_bar_v_sig_5)
  Constant97/1 -> Mux22/3
  cal sig/1(z) -> [sigma_bar_w_sig_1]
  trans to column22/1(y) -> [sigma_bar_w_tilt_squ_1]
  [sigma_bar_w_tilt_squ_3] -> cal sig2/1(x)
  [sigma_bar_w_tilt] -> Abs3/1
  Interpreted MATLAB Function24/1 -> trans to column25/1(x)
  [sigma_bar_w_sig_1] -> cal differentiator/5(sigma_bar_v_sig_1)
  cal differentiator/1(d_sigma_bar_v_hat) -> Integrator2/1
  Constant110/1 -> Mux24/3
  cal sig5/1(z) -> [sigma_bar_w_sig_5]
  [sigma_bar_w_tilt] -> Abs4/1
  Demux2/3 -> sigma_bar_w_tilt/3
  cal sig2/1(z) -> [sigma_bar_w_sig_3]
  Constant112/1 -> Product/1
  Constant/1 -> Mux22/2
  cal differentiator/3(d_d2sigma_bar_v_hat) -> Integrator4/1
  Abs3/1 -> Mux24/1
  trans to column21/1(y) -> [sigma_bar_w_tilt_squ_2]
  Constant99/1 -> Add2/1
  Constant103/1 -> cal differentiator/1(c1)
  Mux19/1 -> Interpreted MATLAB Function24/1
  [sigma_bar_w_tilt_squ_6] -> cal sig3/1(x)
  Constant106/1 -> cal differentiator/3(c3)
  [sigma_bar_w_tilt] -> Abs2/1
  [sigma_bar_w_tilt_squ_2] -> cal sig1/1(x)
  Constant162/1 -> Product/2
  Product/1 -> Add1/2
  [sigma_bar_w_sig_4] -> cal differentiator/8(sigma_bar_v_sig_4)
  [sigma_bar_w_hat] -> Add3/1
  Constant102/1 -> Mux20/2
  Add3/1 -> Demux2/1, [sigma_bar_w_tilt]
  cal differentiator/2(d_dsigma_bar_v_hat) -> Integrator3/1
  [sigma_bar_w_tilt] -> Abs5/1
  [sigma_bar_w_tilt] -> cal sig2/2(y)
  [sigma_bar_w_sig_6] -> cal differentiator/10(sigma_bar_v_sig_6)
  trans to column20/1(y) -> [sigma_bar_w_tilt_squ_5]
  Constant104/1 -> cal differentiator/2(c2)
  Constant101/1 -> Mux20/3
  Mux22/1 -> Interpreted MATLAB Function/1
  Constant163/1 -> Product1/2
  Abs2/1 -> Mux23/1
  Interpreted MATLAB Function21/1 -> trans to column21/1(x)
  Interpreted MATLAB Function23/1 -> trans to column24/1(x)
  Mux23/1 -> Interpreted MATLAB Function22/1
  cal sig3/1(z) -> [sigma_bar_w_sig_6]
  Abs4/1 -> Mux19/1
  trans to column25/1(y) -> [sigma_bar_w_tilt_squ_6]
  Constant113/1 -> cal differentiator/4(chi_t)
  choose sigma_bar_w/1(y) -> Add3/2
  Interpreted MATLAB Function/1 -> trans to column22/1(x)
  Interpreted MATLAB Function20/1 -> trans to column20/1(x)
  Constant108/1 -> Mux23/3
  [sigma_bar_w_sig_2] -> cal differentiator/6(sigma_bar_v_sig_2)
  [sigma_bar_w_tilt] -> cal sig1/2(y)
  [sigma_bar_w_tilt_squ_1] -> cal sig/1(x)
  Constant100/1 -> Product1/1
  Abs1/1 -> Mux21/1
  Demux2/2 -> sigma_bar_w_tilt/2
  Integrator4/1 -> [d2_sigma_bar_w_hat], Out3/1
  [sigma_bar_w_tilt_squ_4] -> cal sig4/1(x)
  Abs5/1 -> Mux20/1
  Constant98/1 -> Mux19/3
  Constant111/1 -> Add1/1
  [sigma_bar_w_tilt] -> cal sig5/2(y)
  Constant109/1 -> Mux23/2
  [sigma_bar_w_tilt] -> Abs/1
  Mux24/1 -> Interpreted MATLAB Function23/1
  [sigma_bar_w_tilt] -> Abs1/1
  [sigma_bar_w_tilt_squ_5] -> cal sig5/1(x)
  Add1/1 -> Mux24/2
  cal sig4/1(z) -> [sigma_bar_w_sig_4]
  Constant161/1 -> Add/2
  [sigma_bar_w_tilt] -> cal sig3/2(y)
  Mux21/1 -> Interpreted MATLAB Function21/1
  Interpreted MATLAB Function22/1 -> trans to column23/1(x)
  Mux20/1 -> Interpreted MATLAB Function20/1
  x/1 -> choose sigma_bar_w/1(x)
  Constant105/1 -> Add/1
  Integrator2/1 -> [sigma_bar_w_hat], Out1/1
  Integrator3/1 -> [d_sigma_bar_w_hat], Out2/1

== matlab function sim_new_traj_only_att_ctrl/Qei dynam agent 1 ==
  data: Qei_vec input; dQei_1 output; wei_vec input
function dQei_1 = fcn(Qei_vec, wei_vec)
%%%% 更新四元数误差微分方程
iiuav = 1;

wei = wei_vec(:,iiuav);
thetaei = Qei_vec(1,iiuav);
qei = Qei_vec(2:4,iiuav);

GammaQei = zeros(4,3);
GammaQei(1,:) = -(qei');
GammaQei(2:4,:) = thetaei*eye(3,3) + cal_askew_mat(qei);
dQei_1 = (1/2)*GammaQei*wei;

end

== matlab function sim_new_traj_only_att_ctrl/cal d_theta_hat1 ==
  data: c1 input; d_ui_hat output; d_dui_hat output; d_d2ui_hat output; c2 input; c3 input; chi_t input; ui_sig_1 input; ui_sig_2 input; ui_sig_3 input; ui_sig_4 input; ui_sig_5 input; ui_sig_6 input; dui_hat input; d2ui_hat input
function [d_ui_hat, d_dui_hat, d_d2ui_hat] = fcn(c1, c2, c3, chi_t, ui_sig_1, ui_sig_2, ui_sig_3, ...
                                                                                        ui_sig_4, ui_sig_5, ui_sig_6, dui_hat, d2ui_hat)
d_d2ui_hat = -chi_t .* c1 * ui_sig_1(:) - (1 - chi_t) .* c1 * ui_sig_2(:);
d_dui_hat = -chi_t .* c2 * ui_sig_3(:) - (1 - chi_t) .* c2 * ui_sig_4(:) + d2ui_hat(:);
d_ui_hat = -chi_t .* c3 * ui_sig_5(:) - (1 - chi_t) .* c3 * ui_sig_6(:) + dui_hat(:);

== matlab function sim_new_traj_only_att_ctrl/cal d_theta_hat2 ==
  data: c1 input; d_ui_hat output; d_dui_hat output; d_d2ui_hat output; c2 input; c3 input; chi_t input; ui_sig_1 input; ui_sig_2 input; ui_sig_3 input; ui_sig_4 input; ui_sig_5 input; ui_sig_6 input; dui_hat input; d2ui_hat input
function [d_ui_hat, d_dui_hat, d_d2ui_hat] = fcn(c1, c2, c3, chi_t, ui_sig_1, ui_sig_2, ui_sig_3, ...
                                                                                        ui_sig_4, ui_sig_5, ui_sig_6, dui_hat, d2ui_hat)
d_d2ui_hat = -chi_t .* c1 * ui_sig_1(:) - (1 - chi_t) .* c1 * ui_sig_2(:);
d_dui_hat = -chi_t .* c2 * ui_sig_3(:) - (1 - chi_t) .* c2 * ui_sig_4(:) + d2ui_hat(:);
d_ui_hat = -chi_t .* c3 * ui_sig_5(:) - (1 - chi_t) .* c3 * ui_sig_6(:) + dui_hat(:);

== matlab function sim_new_traj_only_att_ctrl/cal d_theta_hat3 ==
  data: c1 input; d_ui_hat output; d_dui_hat output; d_d2ui_hat output; c2 input; c3 input; chi_t input; ui_sig_1 input; ui_sig_2 input; ui_sig_3 input; ui_sig_4 input; ui_sig_5 input; ui_sig_6 input; dui_hat input; d2ui_hat input
function [d_ui_hat, d_dui_hat, d_d2ui_hat] = fcn(c1, c2, c3, chi_t, ui_sig_1, ui_sig_2, ui_sig_3, ...
                                                                                        ui_sig_4, ui_sig_5, ui_sig_6, dui_hat, d2ui_hat)
d_d2ui_hat = -chi_t .* c1 * ui_sig_1(:) - (1 - chi_t) .* c1 * ui_sig_2(:);
d_dui_hat = -chi_t .* c2 * ui_sig_3(:) - (1 - chi_t) .* c2 * ui_sig_4(:) + d2ui_hat(:);
d_ui_hat = -chi_t .* c3 * ui_sig_5(:) - (1 - chi_t) .* c3 * ui_sig_6(:) + dui_hat(:);

== matlab function sim_new_traj_only_att_ctrl/cal d_theta_hat4 ==
  data: c1 input; d_ui_hat output; d_dui_hat output; d_d2ui_hat output; c2 input; c3 input; chi_t input; ui_sig_1 input; ui_sig_2 input; ui_sig_3 input; ui_sig_4 input; ui_sig_5 input; ui_sig_6 input; dui_hat input; d2ui_hat input
function [d_ui_hat, d_dui_hat, d_d2ui_hat] = fcn(c1, c2, c3, chi_t, ui_sig_1, ui_sig_2, ui_sig_3, ...
                                                                                        ui_sig_4, ui_sig_5, ui_sig_6, dui_hat, d2ui_hat)
d_d2ui_hat = -chi_t .* c1 * ui_sig_1(:) - (1 - chi_t) .* c1 * ui_sig_2(:);
d_dui_hat = -chi_t .* c2 * ui_sig_3(:) - (1 - chi_t) .* c2 * ui_sig_4(:) + d2ui_hat(:);
d_ui_hat = -chi_t .* c3 * ui_sig_5(:) - (1 - chi_t) .* c3 * ui_sig_6(:) + dui_hat(:);

== matlab function sim_new_traj_only_att_ctrl/process velocity ==
  data: T0 input; T1 input; T2 input; PZ0 input; PZ1 input; R0 input; R1 input; Rx2 input; Ry2 input; Rz2 input; t input; V_init_out output
function V_init_out = fcn(T0, T1, T2, PZ0, PZ1, R0, R1, Rx2, Ry2, Rz2, t)
V_init_out = zeros(3, 1);
if t < T1 + 1e-05
    V_init_out(1, 1) = ( cos( ( 2 * pi * ( t - T0 ) ) / ( T0 - T1 ) ) * ( R0 - R1 ) ) / ( T0 - T1 ) ...
                                    - ( 2 * pi * sin( ( 2 * pi * ( t - T0 ) ) / ( T0 - T1 ) ) * ( R0 + ( ( R0 - R1 ) * ( t - T0 ) ) / ( T0 - T1 ) ) ) / ( T0 - T1 );
    V_init_out(2, 1) = ( sin( ( 2 * pi * ( t - T0 ) ) / ( T0 - T1 ) ) * ( R0 - R1 ) ) / ( T0 - T1 ) ...
                                    + ( 2 * pi * cos( ( 2 * pi * ( t - T0 ) ) / ( T0 - T1 ) ) * ( R0 + ( ( R0 - R1 ) * ( t - T0 ) ) / ( T0 - T1 ) ) ) / ( T0 - T1 );
    V_init_out(3, 1) = ( PZ0 - PZ1 ) / ( T0 - T1 );
else
    V_init_out(1, 1) = ( 2 * Rx2 * pi * sin( ( 2 * pi * ( t - T1 ) ) / ( T1 - T2 ) ) ) / ( T1 - T2 );
    V_init_out(2, 1) = ( 4 * Ry2 * pi * cos( ( 4 * pi * ( t - T1 ) ) / ( T1 - T2 ) ) ) / ( T1 - T2 );
    V_init_out(3, 1) = - ( 4 * Rz2 * pi * cos( ( 4 * pi * ( t - T1 ) ) / ( T1 - T2 ) ) ) / ( T1 - T2 );
end

== matlab function sim_new_traj_only_att_ctrl/cal differentiator d_sigma_bar_w_hat agent 1/cal differentiator ==
  data: c1 input; d_sigma_bar_v_hat output; d_dsigma_bar_v_hat output; d_d2sigma_bar_v_hat output; c2 input; c3 input; chi_t input; sigma_bar_v_sig_1 input; sigma_bar_v_sig_2 input; sigma_bar_v_sig_3 input; sigma_bar_v_sig_4 input; sigma_bar_v_sig_5 input; sigma_bar_v_sig_6 input; d_sigma_bar_v_hat input; d2_sigma_bar_v_hat input
function [d_sigma_bar_v_hat, d_dsigma_bar_v_hat, d_d2sigma_bar_v_hat] = fcn(c1, c2, c3, chi_t, sigma_bar_v_sig_1, sigma_bar_v_sig_2, sigma_bar_v_sig_3, ...
                                                                                                                                                sigma_bar_v_sig_4, sigma_bar_v_sig_5, sigma_bar_v_sig_6, d_sigma_bar_v_hat, d2_sigma_bar_v_hat)
d_d2sigma_bar_v_hat = -chi_t .* c1 * sigma_bar_v_sig_1(:) - (1 - chi_t) .* c1 * sigma_bar_v_sig_2(:);
d_dsigma_bar_v_hat = -chi_t .* c2 * sigma_bar_v_sig_3(:) - (1 - chi_t) .* c2 * sigma_bar_v_sig_4(:) + d2_sigma_bar_v_hat(:);
d_sigma_bar_v_hat = -chi_t .* c3 * sigma_bar_v_sig_5(:) - (1 - chi_t) .* c3 * sigma_bar_v_sig_6(:) + d_sigma_bar_v_hat(:);

== matlab function sim_new_traj_only_att_ctrl/cal differentiator d_sigma_bar_w_hat agent 1/cal sig ==
  data: x input; z output; y input
function z = fcn(x, y)
z = x(:) .* sign(y(:));

== matlab function sim_new_traj_only_att_ctrl/cal differentiator d_sigma_bar_w_hat agent 1/cal sig1 ==
  data: x input; z output; y input
function z = fcn(x, y)
z = x(:) .* sign(y(:));

== matlab function sim_new_traj_only_att_ctrl/cal differentiator d_sigma_bar_w_hat agent 1/cal sig2 ==
  data: x input; z output; y input
function z = fcn(x, y)
z = x(:) .* sign(y(:));

== matlab function sim_new_traj_only_att_ctrl/cal differentiator d_sigma_bar_w_hat agent 1/cal sig3 ==
  data: x input; z output; y input
function z = fcn(x, y)
z = x(:) .* sign(y(:));

== matlab function sim_new_traj_only_att_ctrl/cal differentiator d_sigma_bar_w_hat agent 1/cal sig4 ==
  data: x input; z output; y input
function z = fcn(x, y)
z = x(:) .* sign(y(:));

== matlab function sim_new_traj_only_att_ctrl/cal differentiator d_sigma_bar_w_hat agent 1/cal sig5 ==
  data: x input; z output; y input
function z = fcn(x, y)
z = x(:) .* sign(y(:));

== matlab function sim_new_traj_only_att_ctrl/cal differentiator d_sigma_bar_w_hat agent 1/choose sigma_bar_w ==
  data: x input; y output
function y = fcn(x)
iiuav = 1;
y = x(:,iiuav);

== matlab function sim_new_traj_only_att_ctrl/cal differentiator d_sigma_bar_w_hat agent 1/trans to column20 ==
  data: x input; y output
function y = fcn(x)
y = x(:);

== matlab function sim_new_traj_only_att_ctrl/cal differentiator d_sigma_bar_w_hat agent 1/trans to column21 ==
  data: x input; y output
function y = fcn(x)
y = x(:);

== matlab function sim_new_traj_only_att_ctrl/cal differentiator d_sigma_bar_w_hat agent 1/trans to column22 ==
  data: x input; y output
function y = fcn(x)
y = x(:);

== matlab function sim_new_traj_only_att_ctrl/cal differentiator d_sigma_bar_w_hat agent 1/trans to column23 ==
  data: x input; y output
function y = fcn(x)
y = x(:);

== matlab function sim_new_traj_only_att_ctrl/cal differentiator d_sigma_bar_w_hat agent 1/trans to column24 ==
  data: x input; y output
function y = fcn(x)
y = x(:);

== matlab function sim_new_traj_only_att_ctrl/cal differentiator d_sigma_bar_w_hat agent 1/trans to column25 ==
  data: x input; y output
function y = fcn(x)
y = x(:);

== matlab function sim_new_traj_only_att_ctrl/cal differentiator d_sigma_bar_w_hat agent 2/cal differentiator ==
  data: c1 input; d_sigma_bar_v_hat output; d_dsigma_bar_v_hat output; d_d2sigma_bar_v_hat output; c2 input; c3 input; chi_t input; sigma_bar_v_sig_1 input; sigma_bar_v_sig_2 input; sigma_bar_v_sig_3 input; sigma_bar_v_sig_4 input; sigma_bar_v_sig_5 input; sigma_bar_v_sig_6 input; d_sigma_bar_v_hat input; d2_sigma_bar_v_hat input
function [d_sigma_bar_v_hat, d_dsigma_bar_v_hat, d_d2sigma_bar_v_hat] = fcn(c1, c2, c3, chi_t, sigma_bar_v_sig_1, sigma_bar_v_sig_2, sigma_bar_v_sig_3, ...
                                                                                                                                                sigma_bar_v_sig_4, sigma_bar_v_sig_5, sigma_bar_v_sig_6, d_sigma_bar_v_hat, d2_sigma_bar_v_hat)
d_d2sigma_bar_v_hat = -chi_t .* c1 * sigma_bar_v_sig_1(:) - (1 - chi_t) .* c1 * sigma_bar_v_sig_2(:);
d_dsigma_bar_v_hat = -chi_t .* c2 * sigma_bar_v_sig_3(:) - (1 - chi_t) .* c2 * sigma_bar_v_sig_4(:) + d2_sigma_bar_v_hat(:);
d_sigma_bar_v_hat = -chi_t .* c3 * sigma_bar_v_sig_5(:) - (1 - chi_t) .* c3 * sigma_bar_v_sig_6(:) + d_sigma_bar_v_hat(:);

== matlab function sim_new_traj_only_att_ctrl/cal differentiator d_sigma_bar_w_hat agent 2/cal sig ==
  data: x input; z output; y input
function z = fcn(x, y)
z = x(:) .* sign(y(:));

== matlab function sim_new_traj_only_att_ctrl/cal differentiator d_sigma_bar_w_hat agent 2/cal sig1 ==
  data: x input; z output; y input
function z = fcn(x, y)
z = x(:) .* sign(y(:));

== matlab function sim_new_traj_only_att_ctrl/cal differentiator d_sigma_bar_w_hat agent 2/cal sig2 ==
  data: x input; z output; y input
function z = fcn(x, y)
z = x(:) .* sign(y(:));

== matlab function sim_new_traj_only_att_ctrl/Qei dynam agent 2 ==
  data: Qei_vec input; dQei_2 output; wei_vec input
function dQei_2 = fcn(Qei_vec, wei_vec)
%%%% 更新四元数误差微分方程
iiuav = 2;

wei = wei_vec(:,iiuav);
thetaei = Qei_vec(1,iiuav);
qei = Qei_vec(2:4,iiuav);

GammaQei = zeros(4,3);
GammaQei(1,:) = -(qei');
GammaQei(2:4,:) = thetaei*eye(3,3) + cal_askew_mat(qei);
dQei_2 = (1/2)*GammaQei*wei;

end

== matlab function sim_new_traj_only_att_ctrl/cal differentiator d_sigma_bar_w_hat agent 2/cal sig3 ==
  data: x input; z output; y input
function z = fcn(x, y)
z = x(:) .* sign(y(:));

== matlab function sim_new_traj_only_att_ctrl/cal differentiator d_sigma_bar_w_hat agent 2/cal sig4 ==
  data: x input; z output; y input
function z = fcn(x, y)
z = x(:) .* sign(y(:));

== matlab function sim_new_traj_only_att_ctrl/cal differentiator d_sigma_bar_w_hat agent 2/cal sig5 ==
  data: x input; z output; y input
function z = fcn(x, y)
z = x(:) .* sign(y(:));

== matlab function sim_new_traj_only_att_ctrl/cal differentiator d_sigma_bar_w_hat agent 2/choose sigma_bar_w ==
  data: x input; y output
function y = fcn(x)
iiuav = 2;
y = x(:,iiuav);

== matlab function sim_new_traj_only_att_ctrl/cal differentiator d_sigma_bar_w_hat agent 2/trans to column20 ==
  data: x input; y output
function y = fcn(x)
y = x(:);

== matlab function sim_new_traj_only_att_ctrl/cal differentiator d_sigma_bar_w_hat agent 2/trans to column21 ==
  data: x input; y output
function y = fcn(x)
y = x(:);

== matlab function sim_new_traj_only_att_ctrl/cal differentiator d_sigma_bar_w_hat agent 2/trans to column22 ==
  data: x input; y output
function y = fcn(x)
y = x(:);

== matlab function sim_new_traj_only_att_ctrl/cal differentiator d_sigma_bar_w_hat agent 2/trans to column23 ==
  data: x input; y output
function y = fcn(x)
y = x(:);

== matlab function sim_new_traj_only_att_ctrl/cal differentiator d_sigma_bar_w_hat agent 2/trans to column24 ==
  data: x input; y output
function y = fcn(x)
y = x(:);

== matlab function sim_new_traj_only_att_ctrl/cal differentiator d_sigma_bar_w_hat agent 2/trans to column25 ==
  data: x input; y output
function y = fcn(x)
y = x(:);

== matlab function sim_new_traj_only_att_ctrl/cal differentiator d_sigma_bar_w_hat agent 3/cal differentiator ==
  data: c1 input; d_sigma_bar_v_hat output; d_dsigma_bar_v_hat output; d_d2sigma_bar_v_hat output; c2 input; c3 input; chi_t input; sigma_bar_v_sig_1 input; sigma_bar_v_sig_2 input; sigma_bar_v_sig_3 input; sigma_bar_v_sig_4 input; sigma_bar_v_sig_5 input; sigma_bar_v_sig_6 input; d_sigma_bar_v_hat input; d2_sigma_bar_v_hat input
function [d_sigma_bar_v_hat, d_dsigma_bar_v_hat, d_d2sigma_bar_v_hat] = fcn(c1, c2, c3, chi_t, sigma_bar_v_sig_1, sigma_bar_v_sig_2, sigma_bar_v_sig_3, ...
                                                                                                                                                sigma_bar_v_sig_4, sigma_bar_v_sig_5, sigma_bar_v_sig_6, d_sigma_bar_v_hat, d2_sigma_bar_v_hat)
d_d2sigma_bar_v_hat = -chi_t .* c1 * sigma_bar_v_sig_1(:) - (1 - chi_t) .* c1 * sigma_bar_v_sig_2(:);
d_dsigma_bar_v_hat = -chi_t .* c2 * sigma_bar_v_sig_3(:) - (1 - chi_t) .* c2 * sigma_bar_v_sig_4(:) + d2_sigma_bar_v_hat(:);
d_sigma_bar_v_hat = -chi_t .* c3 * sigma_bar_v_sig_5(:) - (1 - chi_t) .* c3 * sigma_bar_v_sig_6(:) + d_sigma_bar_v_hat(:);

== matlab function sim_new_traj_only_att_ctrl/Qei dynam agent 3 ==
  data: Qei_vec input; dQei_3 output; wei_vec input
function dQei_3 = fcn(Qei_vec, wei_vec)
%%%% 更新四元数误差微分方程
iiuav = 3;

wei = wei_vec(:,iiuav);
thetaei = Qei_vec(1,iiuav);
qei = Qei_vec(2:4,iiuav);

GammaQei = zeros(4,3);
GammaQei(1,:) = -(qei');
GammaQei(2:4,:) = thetaei*eye(3,3) + cal_askew_mat(qei);
dQei_3 = (1/2)*GammaQei*wei;

end

== matlab function sim_new_traj_only_att_ctrl/cal differentiator d_sigma_bar_w_hat agent 3/cal sig ==
  data: x input; z output; y input
function z = fcn(x, y)
z = x(:) .* sign(y(:));

== matlab function sim_new_traj_only_att_ctrl/cal differentiator d_sigma_bar_w_hat agent 3/cal sig1 ==
  data: x input; z output; y input
function z = fcn(x, y)
z = x(:) .* sign(y(:));

== matlab function sim_new_traj_only_att_ctrl/cal differentiator d_sigma_bar_w_hat agent 3/cal sig2 ==
  data: x input; z output; y input
function z = fcn(x, y)
z = x(:) .* sign(y(:));

== matlab function sim_new_traj_only_att_ctrl/cal differentiator d_sigma_bar_w_hat agent 3/cal sig3 ==
  data: x input; z output; y input
function z = fcn(x, y)
z = x(:) .* sign(y(:));

== matlab function sim_new_traj_only_att_ctrl/cal differentiator d_sigma_bar_w_hat agent 3/cal sig4 ==
  data: x input; z output; y input
function z = fcn(x, y)
z = x(:) .* sign(y(:));

== matlab function sim_new_traj_only_att_ctrl/cal differentiator d_sigma_bar_w_hat agent 3/cal sig5 ==
  data: x input; z output; y input
function z = fcn(x, y)
z = x(:) .* sign(y(:));

== matlab function sim_new_traj_only_att_ctrl/cal differentiator d_sigma_bar_w_hat agent 3/choose sigma_bar_w ==
  data: x input; y output
function y = fcn(x)
iiuav = 3;
y = x(:,iiuav);

== matlab function sim_new_traj_only_att_ctrl/cal differentiator d_sigma_bar_w_hat agent 3/trans to column20 ==
  data: x input; y output
function y = fcn(x)
y = x(:);

== matlab function sim_new_traj_only_att_ctrl/cal differentiator d_sigma_bar_w_hat agent 3/trans to column21 ==
  data: x input; y output
function y = fcn(x)
y = x(:);

== matlab function sim_new_traj_only_att_ctrl/Qei dynam agent 4 ==
  data: Qei_vec input; dQei_4 output; wei_vec input
function dQei_4 = fcn(Qei_vec, wei_vec)
%%%% 更新四元数误差微分方程
iiuav = 4;

wei = wei_vec(:,iiuav);
thetaei = Qei_vec(1,iiuav);
qei = Qei_vec(2:4,iiuav);

GammaQei = zeros(4,3);
GammaQei(1,:) = -(qei');
GammaQei(2:4,:) = thetaei*eye(3,3) + cal_askew_mat(qei);
dQei_4 = (1/2)*GammaQei*wei;

end

== matlab function sim_new_traj_only_att_ctrl/cal differentiator d_sigma_bar_w_hat agent 3/trans to column22 ==
  data: x input; y output
function y = fcn(x)
y = x(:);
